simulink model "ModelOfLikeTheWholeThing"  (R2017b)
settings: Solver=ode8  StartTime=0.0  StopTime=5  FixedStep=0.01  RelTol=1e-3
InitFcn:
  | ra = 4;
  | jm = 0.0000218;
  | rm = 0.7/100;
  | dsm = 62.892;
  | kt = 0.138;
  | ke = kt;
  | ms = 0.93;
  | hl = 1.5 / 100;
  | Lr = 24.1 / 100;
  | Lcm = hl / 2 + Lr;
  | ml =0.182;
  | mr = 0.085;
  | rl = 20.125 / 1000;
  | Jp =1/3 * mr * Lr^2 + 1/2*ml*rl^2 + ml * Lcm ^ 2;
  | Dp = 0.007;
  | g = 9.82;
StartFcn:
  | ra = 4;
  | jm = 0.0000218;
  | rm = 0.7/100;
  | dsm = 62.892;
  | kt = 0.138;
  | ke = kt;
  | ms = 0.93;
undefined symbols (not defined in the file): National_Instruments, PCI
libraries: sldrtlib x4
settings Model: Creator=labadmin  LastModifiedBy=labadmin
settings RTWCC: SystemTargetFile=sldrt.tlc  TemplateMakefile=sldrt.tmf  Description=Simulink Desktop Real-Time  RTWCompilerOptimization=on
settings CodeAppCC: MaxIdLength=95
settings SimulinkDesktopRealTimeCC: TargetPreCompLibLocation=C:\Program Files\MATLAB\R2017b\toolbox\sldrt\lib\win64

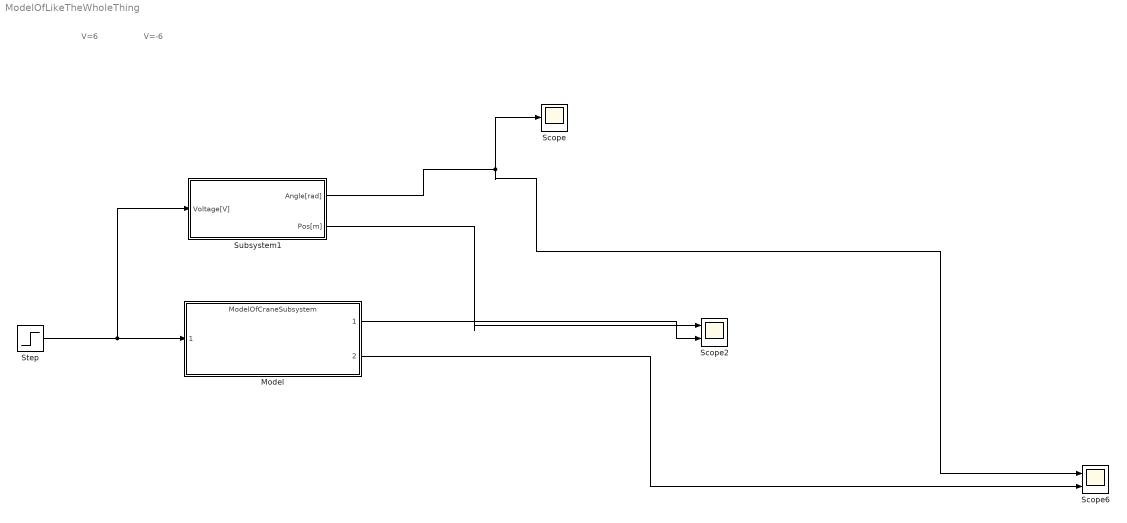
== system ModelOfLikeTheWholeThing ==
  note: V=6
  note: V=-6
  Model : ModelReference  ModelNameDialog=ModelOfCraneSubsystem.slx  SimulationMode=Normal  ModelReferenceVersion=1.3
  Scope : Scope
  Scope2 : Scope  NumInputPorts=2
  Scope6 : Scope  NumInputPorts=2
  Step : Step  Time=2.5  After=0  SampleTime=0
  Subsystem1 : Subsystem
  wires:
  Step/1 -> Subsystem1/1(Voltage[V]), Model/1
  Model/1 -> Scope2/2
  Model/2 -> Scope6/2
  Subsystem1/1(Angle[rad]) -> Scope/1, Scope6/1
  Subsystem1/2(Pos[m]) -> Scope2/1

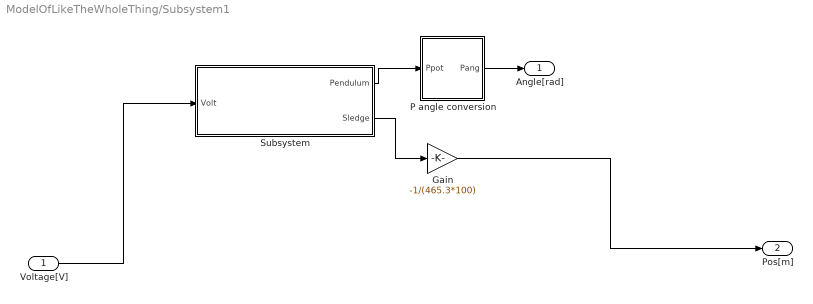
== system ModelOfLikeTheWholeThing/Subsystem1 ==
  Voltage[V] : Inport
  Gain : Gain  Gain=-1/(465.3*100)
  P angle conversion : Subsystem
  Subsystem : Subsystem
  Angle[rad] : Outport
  Pos[m] : Outport  Port=2
  wires:
  Gain/1 -> Pos[m]/1
  P angle conversion/1(Pang) -> Angle[rad]/1
  Subsystem/2(Sledge) -> Gain/1
  Subsystem/1(Pendulum) -> P angle conversion/1(Ppot)
  Voltage[V]/1 -> Subsystem/1(Volt)

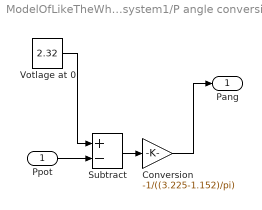
== system ModelOfLikeTheWholeThing/Subsystem1/P angle conversion ==
  Ppot : Inport
  Conversion : Gain  Gain=-1/((3.225-1.152)/pi)
  Subtract : Sum  Inputs=+-
  "Votlage at 0 " : Constant  Value=2.32
  Pang : Outport
  wires:
  Subtract/1 -> Conversion/1
  Ppot/1 -> Subtract/2
  "Votlage at 0 "/1 -> Subtract/1
  Conversion/1 -> Pang/1

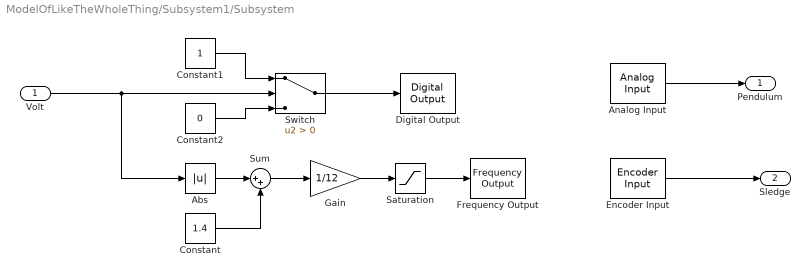
== system ModelOfLikeTheWholeThing/Subsystem1/Subsystem ==
  Volt : Inport
  Abs : Abs
  Analog Input : sldrtlib/Analog Input  SampleTime=-1  MaxMissedTicks=1000000000  ShowMissedTicks=off  YieldWhenWaiting=off  DrvName=National_Instruments/PCI-6229  DrvAddress=4294967295  DrvOptions=[0 1 8192 2 3]  Channels=1  RangeMode=1  VoltRange=1  DataType=1
      settings: AttributesFormatString=National Instruments\nPCI-6229 [auto]  SourceProductName=Simulink Desktop Real-Time
  Constant : Constant  Value=1.4
  Constant1 : Constant
  Constant2 : Constant  Value=0
  Digital Output : sldrtlib/Digital Output  SampleTime=-1  MaxMissedTicks=100000000  ShowMissedTicks=off  YieldWhenWaiting=off  DrvName=National_Instruments/PCI-6229  DrvAddress=4294967295  DrvOptions=[0 1 8192 2 3]  Channels=1  BitMode=1  InitialValue=[]  FinalValue=[]
      settings: AttributesFormatString=National Instruments\nPCI-6229 [auto]  SourceProductName=Simulink Desktop Real-Time  SourceProductBaseCode=WT
  Encoder Input : sldrtlib/Encoder Input  SampleTime=-1  MaxMissedTicks=10000000  ShowMissedTicks=off  YieldWhenWaiting=off  DrvName=National_Instruments/PCI-6229  DrvAddress=4294967295  DrvOptions=[0 1 8192 2 3]  Channels=1  QuadMode=3  IndexPulse=2  InputFilter=Inf  DataType=1
      settings: AttributesFormatString=National Instruments\nPCI-6229 [auto]  SourceProductName=Simulink Desktop Real-Time
  Frequency Output : sldrtlib/Frequency Output  SampleTime=-1  MaxMissedTicks=1000000000  ShowMissedTicks=off  YieldWhenWaiting=off  DrvName=National_Instruments/PCI-6229  DrvAddress=4294967295  DrvOptions=[0 1 8192 2 3]  Channels=2  FrequencySource=1  Frequency=10000  FrequencyFinalValue=[]  DutySource=2  Duty=0  DutyFinalValue=0
      settings: AttributesFormatString=National Instruments\nPCI-6229 [auto]  SourceProductName=Simulink Desktop Real-Time  SourceProductBaseCode=WT
  Gain : Gain  Gain=1/12
  Saturation : Saturate  LowerLimit=0
  Sum : Sum  Inputs=|++
  Switch : Switch  Criteria=u2 > Threshold
  Pendulum : Outport
  Sledge : Outport  Port=2
  wires:
  Analog Input/1 -> Pendulum/1
  Encoder Input/1 -> Sledge/1
  Saturation/1 -> Frequency Output/1
  Volt/1 -> Abs/1, Switch/2
  Gain/1 -> Saturation/1
  Constant2/1 -> Switch/3
  Constant1/1 -> Switch/1
  Switch/1 -> Digital Output/1
  Abs/1 -> Sum/1
  Sum/1 -> Gain/1
  Constant/1 -> Sum/2
